simulink model "dynamic_plaque_model_2021A"  (R2021a)
settings: Solver=FixedStepAuto  StartTime=0.0  StopTime=10.0  RelTol=1e-3
values from neighbouring files (symbols this model uses):
  Fg_sphere = masseS*g    (= 0.07848)    [Constante_L.m]
  Fg_total = masseTotal*g    (= 4.24773)    [Constante_L.m]
  inertiePx = 1.347*10^-3    (= 0.001347)    [Constante_L.m]
  masseTotal = masseP + sig*masseS    (= 0.433)    [Constante_L.m]
  XA = +rABC    (= 0.0952)    [Constante_L.m]
  XB = -rABC*sind(30)    [Constante_L.m]
  XC = -rABC*sind(30)    [Constante_L.m]
  YA = 0.0    (= 0)    [Constante_L.m]
  YB = +rABC*cosd(30)    [Constante_L.m]
  YC = -rABC*cosd(30)    [Constante_L.m]
settings Model: Creator=dupa1607  LastModifiedBy=alexi
settings SolverCC: AlgebraicLoopSolver=TrustRegion
settings DebuggingCC: SFMachineParentedDataDiag=warning

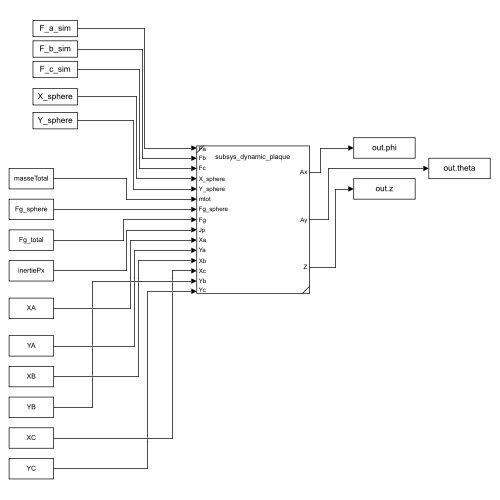
[thumbnail: Simulink's stored preview of the top-level diagram]
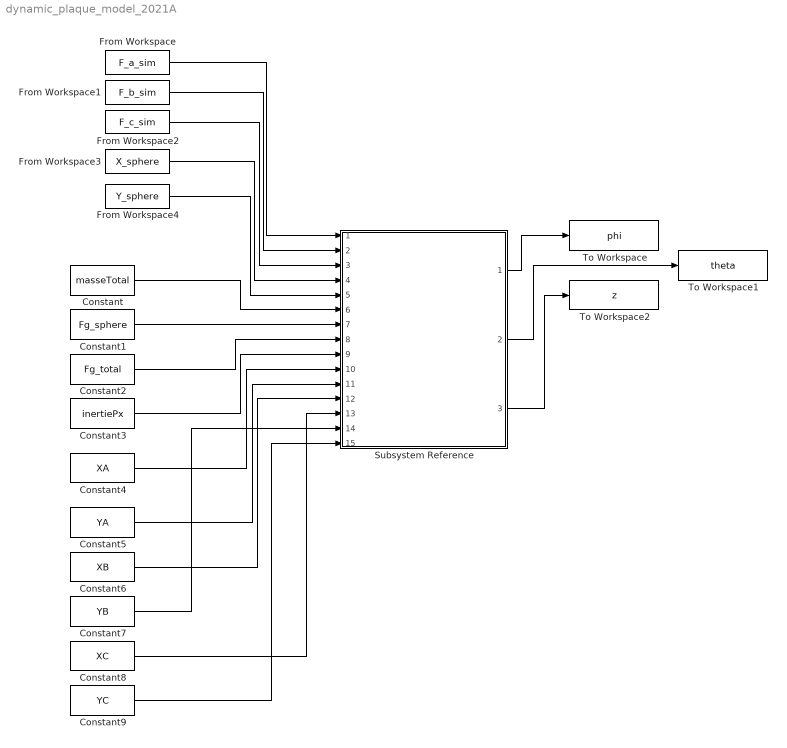
== system dynamic_plaque_model_2021A ==
  Constant : Constant  Value=masseTotal
  Constant1 : Constant  Value=Fg_sphere
  Constant2 : Constant  Value=Fg_total
  Constant3 : Constant  Value=inertiePx
  Constant4 : Constant  Value=XA
  Constant5 : Constant  Value=YA
  Constant6 : Constant  Value=XB
  Constant7 : Constant  Value=YB
  Constant8 : Constant  Value=XC
  Constant9 : Constant  Value=YC
  From Workspace : FromWorkspace  VariableName=F_a_sim
  From Workspace1 : FromWorkspace  VariableName=F_b_sim
  From Workspace2 : FromWorkspace  VariableName=F_c_sim
  From Workspace3 : FromWorkspace  VariableName=X_sphere
  From Workspace4 : FromWorkspace  VariableName=Y_sphere
  Subsystem Reference : Subsystem  ReferencedSubsystem=subsys_dynamic_plaque
  To Workspace : ToWorkspace  VariableName=phi  SaveFormat=Timeseries  SampleTime=-1
  To Workspace1 : ToWorkspace  VariableName=theta  SaveFormat=Timeseries  SampleTime=-1
  To Workspace2 : ToWorkspace  VariableName=z  SaveFormat=Timeseries  SampleTime=-1
  wires:
  From Workspace/1 -> Subsystem Reference/1
  From Workspace1/1 -> Subsystem Reference/2
  From Workspace2/1 -> Subsystem Reference/3
  Subsystem Reference/3 -> To Workspace2/1
  Subsystem Reference/2 -> To Workspace1/1
  Subsystem Reference/1 -> To Workspace/1
  From Workspace3/1 -> Subsystem Reference/4
  From Workspace4/1 -> Subsystem Reference/5
  Constant/1 -> Subsystem Reference/6
  Constant1/1 -> Subsystem Reference/7
  Constant2/1 -> Subsystem Reference/8
  Constant3/1 -> Subsystem Reference/9
  Constant4/1 -> Subsystem Reference/10
  Constant5/1 -> Subsystem Reference/11
  Constant6/1 -> Subsystem Reference/12
  Constant9/1 -> Subsystem Reference/15
  Constant8/1 -> Subsystem Reference/13
  Constant7/1 -> Subsystem Reference/14
